simulink model "HoppingLEGV2"  (Simulink 7.7)
settings: Solver=ode3  StartTime=0.0  StopTime=inf  FixedStep=Td  RelTol=1e-3
values from neighbouring files (symbols this model uses):
  Td = pi/wd    [AnalizaOscilatora.m]    (also in Start.m = 0.001)
libraries: utility x1, vrlib x1
settings Model: Creator=Alan Mutka  LastModifiedBy=Alan Mutka

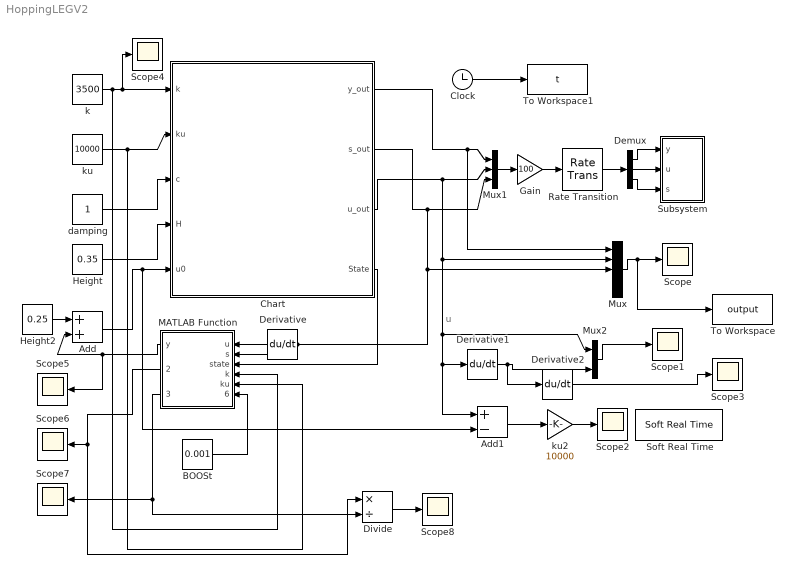
== system HoppingLEGV2 ==
  note: u
  Add : Sum
  Add1 : Sum  Inputs=+-
  BOOSt : Constant  Value=0.001
  Chart : Stateflow chart  TreatAsAtomicUnit=on
  Clock : Clock
      settings: Decimation=10
  Demux : Demux  Outputs=3
  Derivative : Derivative
  Derivative1 : Derivative
  Derivative2 : Derivative
  Divide : Product  Inputs=*/
  Gain : Gain  Gain=100
  Height : Constant  Value=0.35
  Height2 : Constant  Value=0.25
  MATLAB Function : Stateflow chart  TreatAsAtomicUnit=on
  Mux : Mux  Inputs=5
  Mux1 : Mux  Inputs=3
  Mux2 : Mux  Inputs=2
  Rate Transition : RateTransition  OutPortSampleTime=1
  Scope{,1..8} (9 alike) : Scope
      Scope settings: TimeRange=3  YMin=0  YMax=0.55
      Scope1 settings: TimeRange=1.036496350364963  YMin=-2  YMax=1.75
      Scope2 settings: TimeRange=3  YMin=-80  YMax=50  SaveName=ScopeData3
      Scope3 settings: TimeRange=1.036496350364963  YMin=-2  YMax=1.75  SaveName=ScopeData4
      Scope4 settings: TimeRange=3  YMin=2980  YMax=3000  SaveName=ScopeData5
      Scope5 settings: TimeRange=1.036496350364963  YMin=-2  YMax=1.75  SaveName=ScopeData6
      Scope6 settings: TimeRange=1.036496350364963  YMin=2.77556e-017  YMax=0.65  SaveName=ScopeData7
      Scope7 settings: TimeRange=1.036496350364963  YMin=0.045  YMax=0.045  SaveName=ScopeData8
      Scope8 settings: TimeRange=1.036496350364963  YMin=20  YMax=240  SaveName=ScopeData9
  Soft Real Time : utility/Soft Real Time  x=1
  Subsystem : Subsystem
  To Workspace : ToWorkspace  VariableName=output  SampleTime=Td  SaveFormat=Array
  To Workspace1 : ToWorkspace  VariableName=t  SampleTime=Td  SaveFormat=Array
  damping : Constant
  k : Constant  Value=3500
  ku : Constant  Value=10000
  ku2 : Gain  Gain=10000
  wires:
  Clock/1 -> To Workspace1/1
  damping/1 -> Chart/3(c)
  k/1 -> Chart/1(k), Scope4/1, MATLAB Function/4(k)
  Height/1 -> Chart/4(H)
  ku/1 -> Chart/2(ku), MATLAB Function/5(ku)
  Mux/1 -> Scope/1, To Workspace/1
  Chart/1(y_out) -> Mux/1, Mux1/1
  Chart/3(u_out) -> Mux1/2, Mux/2, Mux2/1, Derivative1/1, Add1/1
  Chart/2(s_out) -> Mux/3, Derivative/1, MATLAB Function/2(s), Mux1/3
  Derivative/1 -> MATLAB Function/1(u)
  MATLAB Function/1(y) -> Add/2, Scope5/1
  Mux1/1 -> Gain/1
  Rate Transition/1 -> Demux/1
  Demux/1 -> Subsystem/1(y)
  Demux/2 -> Subsystem/2(u)
  Demux/3 -> Subsystem/3(s)
  Gain/1 -> Rate Transition/1
  Height2/1 -> Add/1
  Chart/4(State) -> MATLAB Function/3(state)
  Mux2/1 -> Scope1/1
  Derivative1/1 -> Mux2/2, Derivative2/1
  Add/1 -> Chart/5(u0), Add1/2
  Add1/1 -> ku2/1
  ku2/1 -> Scope2/1
  Derivative2/1 -> Scope3/1
  BOOSt/1 -> MATLAB Function/6(y_BOOST)
  MATLAB Function/2(E_current) -> Scope6/1, Divide/1
  MATLAB Function/3(E_added) -> Scope7/1, Divide/2
  Divide/1 -> Scope8/1

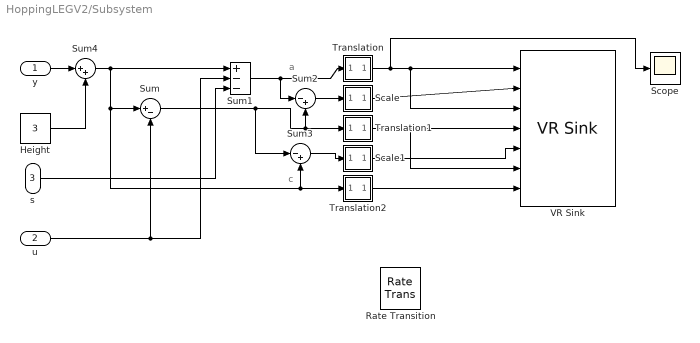
== system HoppingLEGV2/Subsystem ==
  note: c
  note: a
  y : Inport
  u : Inport  Port=2
  s : Inport  Port=3
  Height : Constant  Value=3
  Rate Transition : RateTransition  OutPortSampleTime=0.1
  Scale : Subsystem
  Scale1 : Subsystem
  Scope : Scope
      settings: TimeRange=3  YMin=-4e-015  YMax=4e-015  SaveName=ScopeData2
  Sum : Sum  Inputs=|+-
  Sum1 : Sum  Inputs=|+--
  Sum2 : Sum  Inputs=|-+
  Sum3 : Sum  Inputs=|-+
  Sum4 : Sum  Inputs=|++
  Translation : Subsystem
  Translation1 : Subsystem
  Translation2 : Subsystem
  VR Sink : vrlib/VR Sink  SampleTime=1  ViewEnable=on  RemoteChange=off  RemoteView=on  FieldsWritten=ALFA.translation.3.1.1.double#Opruga.scale.3.1.1.double#Opruga.translation.3.1.1.double#MASS2.translation.3.1.1.double#PRISMATIC.scale.3.1.1.double#PRISMATIC.translation.3.1.1.double#MASS1.translation.3.1.1.double  WorldFileName=skakac2.WRL  AutoView=off  VideoDimensions=[]  FigureProperties="{'Position', 'Name', 'Viewpoint', 'CameraBound', 'CameraDirection', 'CameraPosition', 'CameraUpVector', 'ZoomFactor', 'Antialiasing', 'Headlight', 'Lighting', 'NavPanel', 'StatusBar', 'ToolBar', 'Textures', 'Transparency', 'Wireframe', 'NavZones', 'NavMode', 'NavSpeed', 'Record2DCompressMethod', 'Record2DCompressQuality', 'Record2D', 'Record2DFileName', 'Record2DFPS'; [5.0000000000000000e+000  9.2000000000000000e+001  5.7600000000000000e+002  3.8000000000000000e+002], '', '', 'on', [0.0000000000000000e+000  0.0000000000000000e+000 -1.0000000000000000e+000], [0.0000000000000000e+000  0.0000000000000000e+000  1.1000000000000000e+002], [0.0000000000000000e+000  1.0000000000000000e+000  0.0000000000000000e+000], [1.0000000000000000e+000], 'on', 'on', 'on', 'halfbar', 'on', 'on', 'on', 'on', 'off', 'off', 'fly', 'normal', 'auto', [7.5000000000000000e+001], 'off', '%f_anim_%n.avi', [1.5000000000000000e+001]}"
  wires:
  u/1 -> Sum1/2, Sum/2
  Scale1/1(Out1) -> VR Sink/5
  Sum3/1 -> Scale1/1(In1)
  Sum2/1 -> Scale/1(In1)
  Translation2/1(Out1) -> VR Sink/7
  Translation1/1(Out1) -> VR Sink/6, VR Sink/4
  Scale/1(Out1) -> VR Sink/2
  Translation/1(Out1) -> VR Sink/3, VR Sink/1, Scope/1
  Sum1/1 -> Sum2/1, Translation/1(In1)
  Height/1 -> Sum4/2
  Sum4/1 -> Sum1/1, Sum/1, Translation2/1(In1), Sum3/2
  y/1 -> Sum4/1
  s/1 -> Sum1/3
  Sum/1 -> Translation1/1(In1), Sum2/2, Sum3/1

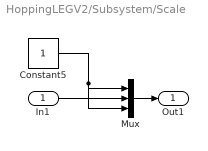
== system HoppingLEGV2/Subsystem/Scale ==
  In1 : Inport
  Constant5 : Constant
  Mux : Mux  Inputs=3
  Out1 : Outport
  wires:
  Constant5/1 -> Mux/3, Mux/1
  In1/1 -> Mux/2
  Mux/1 -> Out1/1

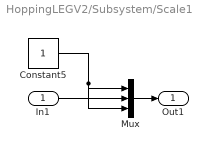
== system HoppingLEGV2/Subsystem/Scale1 ==
  In1 : Inport
  Constant5 : Constant
  Mux : Mux  Inputs=3
  Out1 : Outport
  wires:
  Mux/1 -> Out1/1
  In1/1 -> Mux/2
  Constant5/1 -> Mux/1, Mux/3

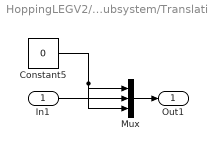
== system HoppingLEGV2/Subsystem/Translation ==
  In1 : Inport
  Constant5 : Constant  Value=0
  Mux : Mux  Inputs=3
  Out1 : Outport
  wires:
  Mux/1 -> Out1/1
  In1/1 -> Mux/2
  Constant5/1 -> Mux/1, Mux/3

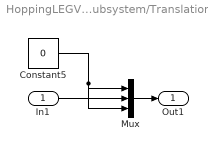
== system HoppingLEGV2/Subsystem/Translation1 ==
  In1 : Inport
  Constant5 : Constant  Value=0
  Mux : Mux  Inputs=3
  Out1 : Outport
  wires:
  Constant5/1 -> Mux/3, Mux/1
  In1/1 -> Mux/2
  Mux/1 -> Out1/1

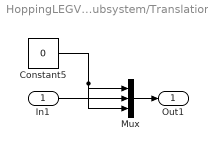
== system HoppingLEGV2/Subsystem/Translation2 ==
  In1 : Inport
  Constant5 : Constant  Value=0
  Mux : Mux  Inputs=3
  Out1 : Outport
  wires:
  Mux/1 -> Out1/1
  In1/1 -> Mux/2
  Constant5/1 -> Mux/1, Mux/3

== stateflow chart Chart ==
  settings: updateMethod=CONTINUOUS
  state Swing
    du:
    y_dot=yv;
    yv_dot=-u*(ku/m1)-g+ku*u0/m1;
    u_dot=uv;
    uv_dot=-u*(ku/m1+ku/m2)+ku*u0/m1+ku*u0/m2;
    //output
    y_out = y;
    s_out=s0;
    u_out=u;
    State=1;
  state Stancedown
    du:
    y_dot = yv;
    yv_dot = ku/m1*(u0-u) -g;
    u_dot=uv;
    uv_dot=k/m2*y+yv*c/m2-u*(ku/m1+k/m2+ku/m2)-uv*c/m2 -k*s0/m2+ku*u0/m1+ku*u0/m2;
    y_out = y;
    s_out=y-u;
    u_out=u;
    State = 0;
  (default) -> Swing : {
      | y=H;yv=0;
      | u=u0_initial;uv=0;
      | }
  Swing -> Stancedown : [y<=l0 && yv<0]
      | {
      |
      |
      |
      | }
  Stancedown -> Swing : [y>l0 && yv>0]
      | {
      |
      |
      |
      | }
  data: yv local double; y_out output double; y local double; k input double =800; ku input double =10000; m1 constant double =1; l0 constant double =0.3; c input double =6; H input double; u local double; uv local double; m2 constant double =0.1; s_out output double; s0 constant double =0.05; g constant double =9.81; u0 input double =4; u_out output double; State output double; u0_initial constant double =0.25
  data yv settings: updateMethod=SF_CONTINUOUS_TIME_DATA
  data y settings: updateMethod=SF_CONTINUOUS_TIME_DATA
  data H settings: updateMethod=SF_CONTINUOUS_TIME_DATA
  data u settings: updateMethod=SF_CONTINUOUS_TIME_DATA
  data uv settings: updateMethod=SF_CONTINUOUS_TIME_DATA

== matlab function MATLAB Function ==
  data: u input double; y output double; s input double; E_current output double; state input double; E_added output double; k input double; ku input double; y_BOOST input double
function [y,E_current,E_added] = fcn(u,s,state,k,ku,y_BOOST)
%#codegen
%#codegen

persistent okidanje;
persistent lastY;
persistent Hout;
persistent Hout_max;
persistent lastState;
persistent last_E_current;
persistent last_E_added;

if isempty(okidanje)
    okidanje = 0;
    lastY = 0;
    Hout=0;
    lastState=state;
    last_E_current =0;
    last_E_added =0;
end

if u > 0
    y=y_BOOST;
    if(y>0 && lastY==0) 
        okidanje=1;
    else
        okidanje=0;
    end
    
    lastY=y;
else 
    y=0;
    lastY=y;
end

if(lastState==1 && state==0)%prije u zraku, sad na zemljim, resetiraj
    Hout=0;
end
lastState=state;

if(okidanje==1 )
    %H=5+ (1/2*abs(1-s)^2*800 + 1/2*0.001^2*10000)/(0.1*9.81)%ovo je bilo
    %prije
    last_E_current=1/2*abs(0.041-s)^2*k;
    last_E_added=1/2*y_BOOST^2*ku;
%     if(H>Hout) 
%         Hout=H;
%     end
end
E_current=last_E_current;
E_added = last_E_added;
